simulink library "posefilter"  (R2019b)
settings: Solver=VariableStepAuto  StartTime=0.0  StopTime=10.0  RelTol=1e-3

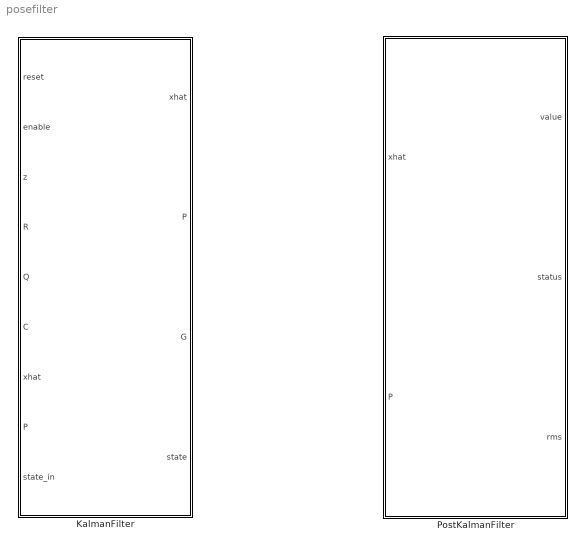
== system posefilter ==
  KalmanFilter : MATLAB Function  TreatAsAtomicUnit=on
  PostKalmanFilter : MATLAB Function  TreatAsAtomicUnit=on

== matlab function posefilter/PostKalmanFilter ==
function [value,status, rms]  = PostKalmanFilter(xhat,P)

value =xhat;
status = SignalState.SIGNALSTATE_UPDATED_;
rms = P;

== matlab function posefilter/KalmanFilter ==
function [xhat,P,G,state]  = KalmanFilter(reset,enable,z,R,Q,C,xhat,P,state_in)
state = state_in;
if(reset == uint8(1))
    state.initialized = uint8(0);
    state.update_counter = uint32(0);
end
if(enable == uint8(1))
    if(state.initialized==0)
        xhat = sum(z)/length(z);
        state.initialized=uint8(1);
        P = 1;
    end
    state.update_counter = state.update_counter+1;

    %Predict Step
    %xhat = xhat; %Notation
    P = P + Q;

    %Update Step
    T = C*P*C'+R;
    G = P*C'*(T^-1);
    P = (1-G*C)*P;
    xhat = xhat + G*(z-(C*xhat));
else
    G = zeros(size(z))';
end
